simulink model "motorlagleadcompensator"  (R2021b)
settings: Solver=VariableStepAuto  StartTime=0.0  StopTime=20  RelTol=1e-3
values from neighbouring files (symbols this model uses):
  b = 0.1    [simscapeParameters.m]    (also in simscapeVisualization.m)
  J = 0.01    [simscapeParameters.m]    (also in simscapeVisualization.m)
  K = 0.01    [simscapeParameters.m]    (also in simscapeVisualization.m)
  L = 0.5    [simscapeParameters.m]    (also in simscapeVisualization.m)
  R = 1    [simscapeParameters.m]    (also in simscapeVisualization.m)
libraries: aerolibanimutils x1
settings Model: Creator=Joshua  LastModifiedBy=Joshua

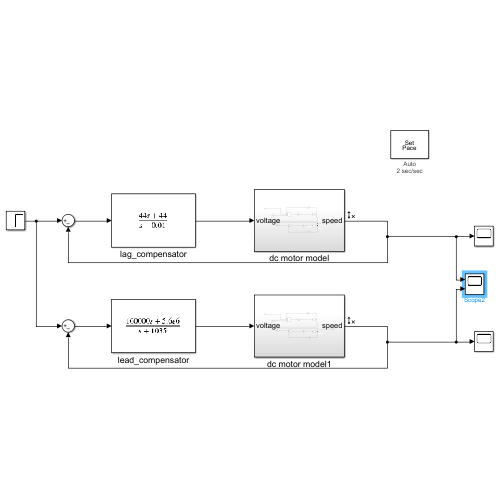
[thumbnail: Simulink's stored preview of the top-level diagram]
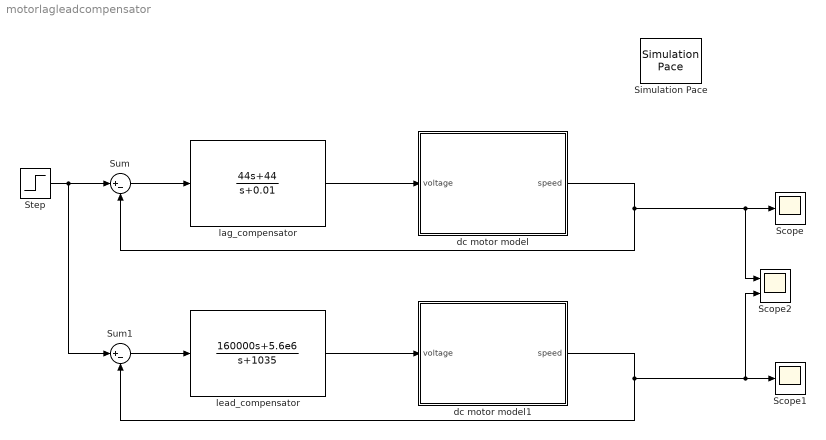
== system motorlagleadcompensator ==
  Scope : Scope
  Scope1 : Scope
  Scope2 : Scope  NumInputPorts=2
  Simulation Pace : aerolibanimutils/Simulation Pace  SimulationPace=2  SleepMode=Auto  OutputPaceError=off  SampleTime=1/30
  Step : Step  SampleTime=0
  Sum : Sum  Inputs=|+-
  Sum1 : Sum  Inputs=|+-
  dc motor model : Subsystem
  dc motor model1 : Subsystem
  lag_compensator : TransferFcn  Numerator=[44 44]  Denominator=[1 0.01]
  lead_compensator : TransferFcn  Numerator=[160000 5.6e6]  Denominator=[1 1035]
  wires:
  dc motor model/1(speed) -> Sum/2, Scope2/1, Scope/1
  Sum/1 -> lag_compensator/1
  lag_compensator/1 -> dc motor model/1(voltage)
  lead_compensator/1 -> dc motor model1/1(voltage)
  dc motor model1/1(speed) -> Sum1/2, Scope2/2, Scope1/1
  Step/1 -> Sum1/1, Sum/1
  Sum1/1 -> lead_compensator/1

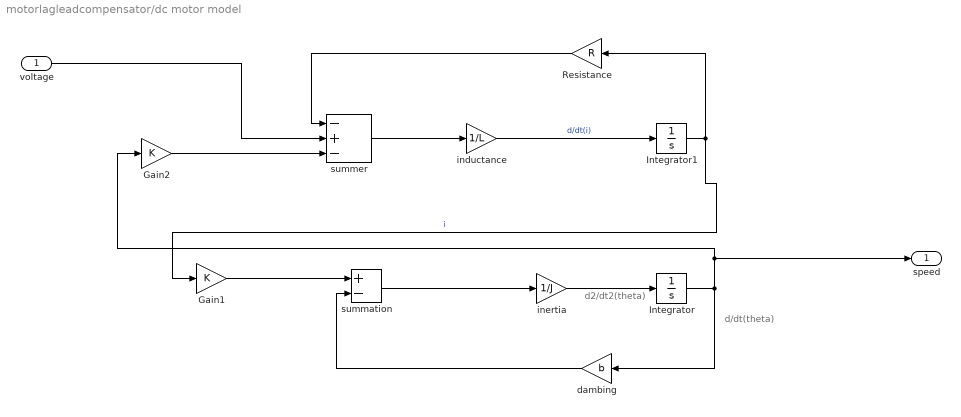
== system motorlagleadcompensator/dc motor model ==
  note: d/dt(theta)
  note: d2/dt2(theta)
  voltage : Inport
  Gain1 : Gain  Gain=K
  Gain2 : Gain  Gain=K
  Integrator : Integrator
  Integrator1 : Integrator
  Resistance : Gain  Gain=R
  dambing : Gain  Gain=b
  inductance : Gain  Gain=1/L
  inertia : Gain  Gain=1/J
  summation : Sum  Inputs=+-
  summer : Sum  Inputs=-+-
  speed : Outport
  wires:
  inductance/1 -> Integrator1/1  "d/dt(i)"
  Integrator1/1 -> Gain1/1, Resistance/1  "i"
  summer/1 -> inductance/1
  summation/1 -> inertia/1
  dambing/1 -> summation/2
  Gain1/1 -> summation/1
  Integrator/1 -> speed/1, Gain2/1, dambing/1
  voltage/1 -> summer/2
  inertia/1 -> Integrator/1
  Resistance/1 -> summer/1
  Gain2/1 -> summer/3

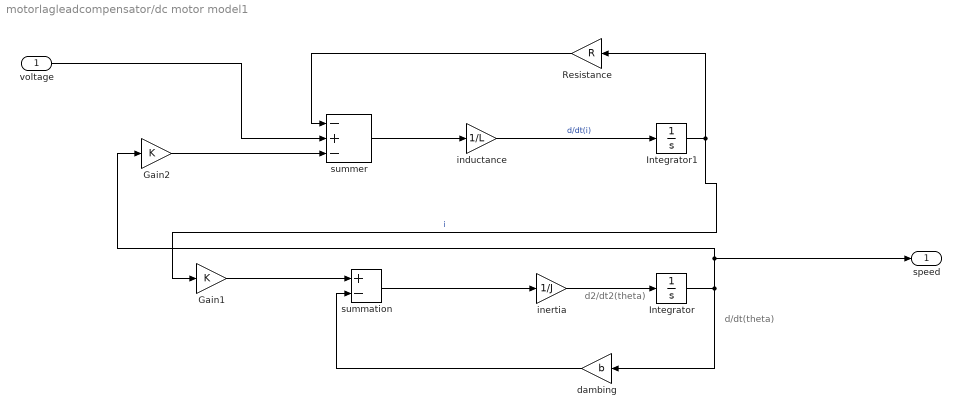
== system motorlagleadcompensator/dc motor model1 ==
  note: d/dt(theta)
  note: d2/dt2(theta)
  voltage : Inport
  Gain1 : Gain  Gain=K
  Gain2 : Gain  Gain=K
  Integrator : Integrator
  Integrator1 : Integrator
  Resistance : Gain  Gain=R
  dambing : Gain  Gain=b
  inductance : Gain  Gain=1/L
  inertia : Gain  Gain=1/J
  summation : Sum  Inputs=+-
  summer : Sum  Inputs=-+-
  speed : Outport
  wires:
  inductance/1 -> Integrator1/1  "d/dt(i)"
  Integrator1/1 -> Gain1/1, Resistance/1  "i"
  summer/1 -> inductance/1
  summation/1 -> inertia/1
  dambing/1 -> summation/2
  Gain1/1 -> summation/1
  Integrator/1 -> speed/1, Gain2/1, dambing/1
  voltage/1 -> summer/2
  inertia/1 -> Integrator/1
  Resistance/1 -> summer/1
  Gain2/1 -> summer/3
